simulink model "A320_23b"  (R2023b)
settings: Solver=ode4  StartTime=0.0  StopTime=150  FixedStep=0.001  RelTol=1e-3
InitFcn:
  | % 清空工作区
  | % clear;
  | 
  | % 加载气动数据
  | load('engine_ct_table.mat'); % 或者是你那个存有气动数据的文件名
values from neighbouring files (symbols this model uses):
  a0 = 340.294    [basedata.m]    (also in basedata.mat; control_design.mat; landing_init.m; landing_plan.mat)
  b_ref = 2.0    (= 2)    [basedata.m]    (also in basedata.mat; control_design.mat; landing_init.m; landing_plan.mat)
  c_gear = [0.8e4, 1.4e4, 1.4e4]    [basedata.m]    (also in basedata.mat = [8000 14000 14000]; control_design.mat = [8000 14000 14000]; landing_init.m; landing_plan.mat = [8000 14000 14000])
  c_lat = [1.4e4, 2.2e4, 2.2e4]    [basedata.m]    (also in basedata.mat = [14000 22000 22000]; control_design.mat = [14000 22000 22000]; landing_init.m; landing_plan.mat = [14000 22000 22000])
  c_ref = 0.9    [basedata.m]    (also in basedata.mat; control_design.mat; landing_init.m; landing_plan.mat)
  c_roll = [0.020, 0.018, 0.018]    [basedata.m]    (also in basedata.mat = [0.02 0.018 0.018]; control_design.mat = [0.02 0.018 0.018]; landing_init.m; landing_plan.mat = [0.02 0.018 0.018])
  CD0 = 0.045    [basedata.m]    (also in basedata.mat; canshujisuan.m; control_design.mat; landing_init.m)
  Clb = -0.08    [basedata.m]    (also in basedata.mat; control_design.mat; landing_init.m; landing_plan.mat)
  Clda = -0.20    (= -0.2)    [basedata.m]    (also in basedata.mat; control_design.mat; landing_init.m; landing_plan.mat)
  CLde = 0.28    [basedata.m]    (also in basedata.mat; control_design.mat; landing_init.m; landing_plan.mat)
  Clp = -0.70    (= -0.7)    [basedata.m]    (also in basedata.mat; control_design.mat; landing_init.m; landing_plan.mat)
  CLq = 4.50    (= 4.5)    [basedata.m]    (also in basedata.mat; canshujisuan.m = 3; control_design.mat; landing_init.m)
  Clr = 0.08    [basedata.m]    (also in basedata.mat; control_design.mat; landing_init.m; landing_plan.mat)
  Cmde = -0.90    (= -0.9)    [basedata.m]    (also in basedata.mat; control_design.mat; landing_init.m; landing_plan.mat)
  Cmq = -18.0    (= -18)    [basedata.m]    (also in basedata.mat; control_design.mat; landing_init.m; landing_plan.mat)
  Cnb = 0.25    [basedata.m]    (also in basedata.mat; control_design.mat; landing_init.m; landing_plan.mat)
  Cndr = -0.15    [basedata.m]    (also in basedata.mat; control_design.mat; landing_init.m; landing_plan.mat)
  Cnp = -0.04    [basedata.m]    (also in basedata.mat; control_design.mat; landing_init.m; landing_plan.mat)
  Cnr = -0.45    [basedata.m]    (also in basedata.mat; control_design.mat; landing_init.m; landing_plan.mat)
  CSb = -0.70    (= -0.7)    [basedata.m]    (also in basedata.mat; control_design.mat; landing_init.m; landing_plan.mat)
  CSdr = 0.18    [basedata.m]    (also in basedata.mat; control_design.mat; landing_init.m; landing_plan.mat)
  CSr = 0.12    [basedata.m]    (also in basedata.mat; control_design.mat; landing_init.m; landing_plan.mat)
  D = 0.5 * rho0 * V^2 * S_ref * CD_current    [canshujisuan.m]
  D0 = 1400    [basedata.m]    (also in basedata.mat; control_design.mat = 800; landing.m; landing_init.m)
  da_max = 25    [basedata.m]    (also in basedata.mat; control_design.mat; landing_init.m; landing_plan.mat)
  da_min = -da_max    (= -25)    [basedata.m]    (also in basedata.mat; control_design.mat; landing_init.m; landing_plan.mat)
  de_max = 25    [basedata.m]    (also in basedata.mat; control_design.mat; landing_init.m; landing_plan.mat)
  de_min = -de_max    (= -25)    [basedata.m]    (also in basedata.mat; control_design.mat; landing_init.m; landing_plan.mat)
  DH = pi / 180    (= 0.0174532925199)    [basedata.m]    (also in basedata.mat; control_design.mat; landing_init.m; landing_plan.mat)
  dr_max = 25    [basedata.m]    (also in basedata.mat; control_design.mat; landing_init.m; landing_plan.mat)
  dr_min = -dr_max    (= -25)    [basedata.m]    (also in basedata.mat; control_design.mat; landing_init.m; landing_plan.mat)
  g = 9.80665    [basedata.m]    (also in basedata.mat; canshujisuan.m; control_design.mat; landing_init.m)
  ground_z = 0.0    (= 0)    [basedata.m]    (also in basedata.mat; control_design.mat; landing_init.m; landing_plan.mat)
  H_B = 132.622761894    [basedata.mat]    (also in landing_trajectory.m = H_R - R * cos(a1); landingplan.mat)
  H_C = 72.1000994005    [basedata.mat]    (also in landing_trajectory.m = H_R - R * cos(a2); landingplan.mat)
  H_climb_complete = 1000    [control_design.mat]    (also in landing.m; landing_init.m; landing_plan.mat; landingplan.mat)
  H_entry = 1000    [basedata.mat]    (also in landing_trajectory.m; landingplan.mat)
  H_exp = 20    [basedata.mat]    (also in landing_trajectory.m; landingplan.mat)
  HD = 180 / pi    (= 57.2957795131)    [basedata.m]    (also in basedata.mat; control_design.mat; landing_init.m; landing_plan.mat)
  I = [ Ixx, -Ixy, -Ixz ... (first row only)    [basedata.m]    (also in basedata.mat = [120  0  0; 0  480  0; 0  0  520]; control_design.mat = [120  0  0; 0  480  0; 0  0  520]; landing_init.m; landing_plan.mat = [120  0  0; 0  480  0; 0  0  520])
  K_alpha = 7.5375    [basedata.mat]    (also in control_design.m = (((wd_pitch^2)-a24))/(2*kesi_pitch*wd_pitch); control_design.mat; controller.m = 5; landingplan.mat)
  k_gear = [1.0e5, 3.0e5, 3.0e5]    [basedata.m]    (also in basedata.mat = [100000 300000 300000]; control_design.mat = [100000 300000 300000]; landing_init.m; landing_plan.mat = [100000 300000 300000])
  Kn_pitch = -0.120095403309    [basedata.mat]    (also in control_design.m = -(2.2*g*(wd_pitch)^2)/(Tr*(((wd_pitch)^2)-a24)*V_control*a34; control_design.mat; controller.m = (2.2*wd^2*g)/(Tr*(wd^2-a24)*V_test*a34); landingplan.mat)
  Kw_pitch = -0.483749055178    [basedata.mat]    (also in control_design.m = -2*kesi_pitch*wd_pitch/a25; control_design.mat; controller.m = -(2*zeta*wd) / a25; landingplan.mat)
  m = 600.0    (= 600)    [basedata.m]    (also in basedata.mat; canshujisuan.m; control_design.mat; landing_init.m)
  mu_brake = [0.0, 0.55, 0.55]    [basedata.m]    (also in basedata.mat = [0 0.55 0.55]; control_design.mat = [0 0.55 0.55]; landing_init.m; landing_plan.mat = [0 0.55 0.55])
  phi0 = 0    [control_design.mat]    (also in landing.m; landing_init.m; landing_init.mat; landing_plan.mat)
  psi0 = 0    [control_design.mat]    (also in landing.m; landing_init.m; landing_init.mat; landing_plan.mat)
  r_left_b = r_gear_b(:,2)    [basedata.m]    (also in basedata.mat = [-0.333333333333 -0.8 0.65]; control_design.mat = [-0.333333333333 -0.8 0.65]; landing_init.m; landing_plan.mat = [-0.333333333333 -0.8 0.65])
  r_nose_b = r_gear_b(:,1)    [basedata.m]    (also in basedata.mat = [2 0 0.65]; control_design.mat = [2 0 0.65]; landing_init.m; landing_plan.mat = [2 0 0.65])
  r_right_b = r_gear_b(:,3)    [basedata.m]    (also in basedata.mat = [-0.333333333333 0.8 0.65]; control_design.mat = [-0.333333333333 0.8 0.65]; landing_init.m; landing_plan.mat = [-0.333333333333 0.8 0.65])
  rho0 = 1.225    [basedata.m]    (also in basedata.mat; canshujisuan.m; control_design.mat; landing_init.m)
  S_ref = 1.2    [basedata.m]    (also in basedata.mat; canshujisuan.m; control_design.mat; landing_init.m)
  theta0 = 0    [control_design.mat]    (also in landing.m; landing_init.m; landing_init.mat = 0.0523598775598; landing_plan.mat = 0.0523560209424)
  V_app = 128.516392565    [basedata.mat]    (also in landing_trajectory.m = 1.4 * Vs; landingplan.mat)
  V_cruise = 200    [basedata.m]
  v_eps = 0.20    (= 0.2)    [basedata.m]    (also in basedata.mat; control_design.mat; landing_init.m; landing_plan.mat)
  V_flare = V_shallow    [landing_trajectory.m]
  V_min = 3    [control_design.mat]    (also in landing.m; landing_init.m; landing_plan.mat; landingplan.mat)
  V_shallow = 110.156907913    [basedata.mat]    (also in landing_trajectory.m = 1.2 * Vs; landingplan.mat)
  wheel_radius = 0.18    [basedata.m]    (also in basedata.mat; control_design.mat; landing_init.m; landing_plan.mat)
  WOW_on = 0.000    (= 0)    [basedata.m]    (also in basedata.mat; control_design.mat; landing_init.m; landing_plan.mat)
  Xg0 = 0    [control_design.mat]    (also in landing.m = -12000; landing_init.m = -12000; landing_init.mat = -8000; landing_plan.mat = -12000)
  Yg0 = 3    [control_design.mat]    (also in landing.m = 0; landing_init.m = 0; landing_init.mat = 0; landing_plan.mat = 0)
  Zg0 = ground_z - wheel_radius - r_gear_b(3,1) + static_deflection    [basedata.m]    (also in basedata.mat = -0.8215943; control_design.mat = -0.8215943; landing.m = -1000; landing_init.m = -1000)
undefined symbols (not defined in the file or in its folder): alpha_CL_table, alpha_Cm_table, alpha_Kde_table, CL_D0, CL_table, Cldr, Cm_table, Cnda, CT_ref, CT_table, CYp, Delta_CD_flap_tot, Delta_CD_gear, Delta_CD_sp, Delta_CL_flap_tot, Delta_CL_sp, Delta_Cm_flap_tot, Delta_Cm_gear, Delta_Cm_sp, delta_flap_TE_max, delta_flap_TE_tab, delta_slat_LE_max, delta_slat_LE_tab, gD_flap_TE_tab, gD_slat_LE_tab, gL_flap_TE_tab, gL_slat_LE_tab, I_xz, I_yz, Ix_Iy, Iy_Iz, Iz_Ix, K_GE, k_i_eff, Kde_table, Mach, N1, N1_idle, N1_lim, spoiler_max_air, T_static, X_landing_start
libraries: simulink x51, matrix_library x19
(part 2 of 4)

== system A320_23b/6DOF-MODEL/AERO-PARAMETER/atmosphere ==
  Add : Sum
  Band-Limited White Noise : simulink/Sources/Band-Limited White Noise  Cov=[1]  Ts=0.1  seed=[23341]
  Constant1 : Constant  Value=rho0
  Constant2 : Constant  Value=a0
  Constant3 : Constant  Value=0.5
  Constant4 : Constant  Value=0
  Constant5 : Constant  Value=0
  Constant6 : Constant  Value=5
  Display : Display
  Gain : Gain
  MATLAB Function : MATLAB Function  TreatAsAtomicUnit=on
  Matrix Multiply : Product  Multiplication=Matrix(*)
  Mux : Mux  Inputs=3
  Product : Product  Inputs=3
  Reshape : Reshape  OutputDimensionality=Column vector (2-D)
  Scope : Scope
  Square : Math  Operator=square
  Transfer Fcn : TransferFcn  Denominator=[10 1]
  tag scope: Vwind_body=global, Vwind_ground=global, a_sound=global, qc=global, rho=global
  wires:
  Constant1/1 -> [rho]
  Constant2/1 -> [a_sound]
  Constant3/1 -> Product/1
  [rho] -> Product/2
  Product/1 -> Display/1, [qc]
  Square/1 -> Product/3
  [Vg] -> Square/1
  Reshape/1 -> [Vwind_ground]
  [Vwind_ground] -> Matrix Multiply/2
  [theta_eular] -> MATLAB Function/2(theta)
  [phi_eular] -> MATLAB Function/1(phi)
  MATLAB Function/1(R_bg) -> Matrix Multiply/1
  [psi_eular] -> MATLAB Function/3(psi)
  Matrix Multiply/1 -> [Vwind_body]
  Gain/1 -> Add/1
  Transfer Fcn/1 -> Gain/1
  Band-Limited White Noise/1 -> Transfer Fcn/1
  Constant5/1 -> Mux/3
  Constant4/1 -> Mux/1
  Add/1 -> Scope/1, Mux/2
  Constant6/1 -> Add/2

== system A320_23b/6DOF-MODEL/AERO-PARAMETER/侧向力系数 ==
  beta(H) : Inport
  dr(H) : Inport  Port=2
  Add : Sum  Inputs=++++
  CYpConst : Constant  Value=CYp
  CYpXPhat : Product
  Constant1 : Constant  Value=CSb
  Constant2 : Constant  Value=CSr
  Constant3 : Constant  Value=CSdr
  Product : Product
  Product2 : Product
  Product3 : Product
  CS : Outport
  wires:
  Add/1 -> CS/1
  Constant3/1 -> Product2/2
  Product2/1 -> Add/3
  dr(H)/1 -> Product2/1
  beta(H)/1 -> Product/1
  Constant1/1 -> Product/2
  Constant2/1 -> Product3/2
  [r_hat] -> Product3/1
  Product/1 -> Add/1
  Product3/1 -> Add/2
  [p_hat] -> CYpXPhat/1
  CYpConst/1 -> CYpXPhat/2
  CYpXPhat/1 -> Add/4

== system A320_23b/6DOF-MODEL/AERO-PARAMETER/俯仰力矩系数 ==
  alpha(H) : Inport
  de(H) : Inport  Port=2
  delta_flap_TE : Inport  Port=3
  delta_slat_LE : Inport  Port=4
  delta_spL : Inport  Port=5
  delta_spR : Inport  Port=6
  eta_gear : Inport  Port=7
  Add : Sum  Inputs=++++++
  CmdeXKde : Product
  Constant1 : Lookup_n-D  NumberOfTableDimensions=1  BreakpointsForDimension1=alpha_Cm_table  Table=Cm_table  InterpMethod=Akima spline
  Constant2 : Constant  Value=Cmq
  Constant3 : Constant  Value=Cmde
  FlapMSum : Sum  Inputs=|++
  FlapMTotal : Gain  Gain=Delta_Cm_flap_tot
  Gain : Gain  Gain=-1
  GearMTotal : Gain  Gain=Delta_Cm_gear
  KdeLookup : Lookup_n-D  NumberOfTableDimensions=1  BreakpointsForDimension1=alpha_Kde_table  Table=Kde_table  InterpMethod=Akima spline
  LENorm : Gain  Gain=1/delta_slat_LE_max
  Product2 : Product
  Product3 : Product
  SpMEta : Gain  Gain=1/(2*spoiler_max_air)
  SpMSum : Sum  Inputs=|++
  SpMTotal : Gain  Gain=Delta_Cm_sp
  TENorm : Gain  Gain=1/delta_flap_TE_max
  Cm : Outport
  wires:
  de(H)/1 -> Product2/1
  Add/1 -> Cm/1
  Constant2/1 -> Product3/2
  [q_hat] -> Product3/1
  Product3/1 -> Add/3
  alpha(H)/1 -> KdeLookup/1, Constant1/1
  Constant3/1 -> CmdeXKde/1
  KdeLookup/1 -> CmdeXKde/2
  CmdeXKde/1 -> Product2/2
  Constant1/1 -> Gain/1
  delta_flap_TE/1 -> TENorm/1
  delta_slat_LE/1 -> LENorm/1
  TENorm/1 -> FlapMSum/1
  LENorm/1 -> FlapMSum/2
  FlapMSum/1 -> FlapMTotal/1
  FlapMTotal/1 -> Add/5
  delta_spL/1 -> SpMSum/1
  delta_spR/1 -> SpMSum/2
  SpMSum/1 -> SpMEta/1
  SpMEta/1 -> SpMTotal/1
  SpMTotal/1 -> Add/6
  eta_gear/1 -> GearMTotal/1
  GearMTotal/1 -> Add/4
  Product2/1 -> Add/2
  Gain/1 -> Add/1

== system A320_23b/6DOF-MODEL/AERO-PARAMETER/偏航力矩系数 ==
  beta(H) : Inport
  dr(H) : Inport  Port=2
  da(H) : Inport  Port=3
  Add : Sum  Inputs=+++++
  CndaConst : Constant  Value=Cnda
  CndaXDa : Product
  Constant1 : Constant  Value=Cnb
  Constant2 : Constant  Value=Cnp
  Constant3 : Constant  Value=Cndr
  Constant4 : Constant  Value=Cnr
  Product{,1..3} (4 alike) : Product
  Cn : Outport
  wires:
  Product2/1 -> Add/4
  Constant4/1 -> Product1/2
  Product/1 -> Add/1
  dr(H)/1 -> Product2/1
  Constant3/1 -> Product2/2
  beta(H)/1 -> Product/1
  Constant1/1 -> Product/2
  Add/1 -> Cn/1
  Constant2/1 -> Product3/2
  [p_hat] -> Product3/1
  Product1/1 -> Add/3
  [r_hat] -> Product1/1
  Product3/1 -> Add/2
  da(H)/1 -> CndaXDa/1
  CndaConst/1 -> CndaXDa/2
  CndaXDa/1 -> Add/5

== system A320_23b/6DOF-MODEL/AERO-PARAMETER/力矩系数2力矩 ==
  Cl/Cm/Cn : Inport
  Constant : Constant  Value=S_ref
  Constant1 : Constant  Value=c_ref
  Constant2 : Constant  Value=b_ref
  Demux : Demux  Outputs=3
  Mux : Mux  Inputs=3
  Product : Product  Inputs=4
  Product1 : Product  Inputs=4
  Product2 : Product  Inputs=4
  MX/MY/MZ : Outport
  wires:
  Cl/Cm/Cn/1 -> Demux/1
  Demux/1 -> Product/1
  Constant/1 -> Product/2, Product1/2, Product2/2
  Demux/3 -> Product2/1
  Demux/2 -> Product1/1
  [qc] -> Product/3, Product2/3, Product1/3
  Product/1 -> Mux/1
  Product1/1 -> Mux/2
  Product2/1 -> Mux/3
  Mux/1 -> MX/MY/MZ/1
  Constant2/1 -> Product/4, Product2/4
  Constant1/1 -> Product1/4

== system A320_23b/6DOF-MODEL/AERO-PARAMETER/力系数2力 ==
  CD/CL/CS : Inport
  Constant : Constant  Value=S_ref
  Demux : Demux  Outputs=3
  Display : Display
  Display1 : Display
  Display2 : Display
  Gain : Gain  Gain=-1
  Gain1 : Gain  Gain=-1
  Mux : Mux  Inputs=3
  Product : Product  Inputs=3
  Product1 : Product  Inputs=3
  Product2 : Product  Inputs=3
  D/L/S : Outport
  wires:
  CD/CL/CS/1 -> Demux/1
  Demux/1 -> Product/1
  Constant/1 -> Product2/2, Product1/2, Product/2
  Demux/3 -> Product2/1
  Demux/2 -> Product1/1
  [qc] -> Product2/3, Product1/3, Product/3
  Product/1 -> Display/1, Gain/1
  Product1/1 -> Display1/1, Gain1/1
  Product2/1 -> Display2/1, Mux/3
  Mux/1 -> D/L/S/1
  Gain/1 -> Mux/1
  Gain1/1 -> Mux/2

== system A320_23b/6DOF-MODEL/AERO-PARAMETER/升力系数 ==
  alpha(H) : Inport
  de(H) : Inport  Port=2
  delta_flap_TE : Inport  Port=3
  delta_slat_LE : Inport  Port=4
  delta_spL : Inport  Port=5
  delta_spR : Inport  Port=6
  Add : Sum  Inputs=+++++
  Constant1 : Lookup_n-D  NumberOfTableDimensions=1  BreakpointsForDimension1=alpha_CL_table  Table=CL_table  InterpMethod=Akima spline
  Constant2 : Constant  Value=CLq
  Constant3 : Constant  Value=CLde
  FlapSum : Sum  Inputs=|++
  FlapTotal : Gain  Gain=Delta_CL_flap_tot
  GLLELkup : Lookup_n-D  NumberOfTableDimensions=1  BreakpointsForDimension1=delta_slat_LE_tab  Table=gL_slat_LE_tab  InterpMethod=Akima spline
  GLTELkup : Lookup_n-D  NumberOfTableDimensions=1  BreakpointsForDimension1=delta_flap_TE_tab  Table=gL_flap_TE_tab  InterpMethod=Akima spline
  KGEGain : Gain  Gain=K_GE
  Product2 : Product
  Product3 : Product
  SlatW : Gain  Gain=0.01
  SpEta : Gain  Gain=1/(2*spoiler_max_air)
  SpSum : Sum  Inputs=|++
  SpTotal : Gain  Gain=Delta_CL_sp
  CL : Outport
  tag scope: CLa=global
  wires:
  [q_hat] -> Product3/1
  Constant2/1 -> Product3/2
  de(H)/1 -> Product2/1
  Constant3/1 -> Product2/2
  Product2/1 -> Add/4
  Product3/1 -> Add/3
  alpha(H)/1 -> Constant1/1
  Constant1/1 -> [CLa], Add/1
  Add/1 -> KGEGain/1
  KGEGain/1 -> CL/1
  delta_flap_TE/1 -> GLTELkup/1
  delta_slat_LE/1 -> GLLELkup/1
  GLTELkup/1 -> FlapSum/1
  GLLELkup/1 -> SlatW/1
  SlatW/1 -> FlapSum/2
  FlapSum/1 -> FlapTotal/1
  delta_spL/1 -> SpSum/1
  delta_spR/1 -> SpSum/2
  SpSum/1 -> SpEta/1
  SpEta/1 -> SpTotal/1
  FlapTotal/1 -> Add/2
  SpTotal/1 -> Add/5

== system A320_23b/6DOF-MODEL/AERO-PARAMETER/无量纲化角速率 ==
  p : Inport
  q : Inport  Port=2
  r : Inport  Port=3
  Constant : Constant  Value=V_min
  Max : MinMax  Function=max  Inputs=2
  Scope : Scope
  Subsystem : Subsystem
  Subsystem1 : Subsystem
  Subsystem2 : Subsystem
  tag scope: Va_safe=global, p_hat=global, q_hat=global, r_hat=global
  wires:
  p/1 -> Subsystem2/1(p)
  [Va_safe] -> Subsystem2/2(Va), Subsystem1/2(Va), Subsystem/2(Va)
  Subsystem/1(r_hat) -> [r_hat]
  Subsystem1/1(q_hat) -> Scope/1, [q_hat]
  Subsystem2/1(p_hat) -> [p_hat]
  [Va] -> Max/2
  Constant/1 -> Max/1
  Max/1 -> [Va_safe]
  r/1 -> Subsystem/1(r)
  q/1 -> Subsystem1/1(q)

== system A320_23b/6DOF-MODEL/AERO-PARAMETER/滚转力矩系数 ==
  beta(H) : Inport
  da(H) : Inport  Port=2
  dr(H) : Inport  Port=3
  Add : Sum  Inputs=+++++
  CldrConst : Constant  Value=Cldr
  CldrXDr : Product
  Constant1 : Constant  Value=Clb
  Constant2 : Constant  Value=Clp
  Constant3 : Constant  Value=Clda
  Constant4 : Constant  Value=Clr
  Product{,1..3} (4 alike) : Product
  Cl : Outport
  wires:
  Product3/1 -> Add/2
  da(H)/1 -> Product2/1
  Product/1 -> Add/1
  beta(H)/1 -> Product/1
  Add/1 -> Cl/1
  Constant1/1 -> Product/2
  Constant3/1 -> Product2/2
  Constant2/1 -> Product3/2
  [p_hat] -> Product3/1
  Product1/1 -> Add/3
  [r_hat] -> Product1/1
  Constant4/1 -> Product1/2
  Product2/1 -> Add/4
  dr(H)/1 -> CldrXDr/1
  CldrConst/1 -> CldrXDr/2
  CldrXDr/1 -> Add/5

== system A320_23b/6DOF-MODEL/AERO-PARAMETER/阻力系数 ==
  delta_flap_TE : Inport
  delta_slat_LE : Inport  Port=2
  delta_spL : Inport  Port=3
  delta_spR : Inport  Port=4
  eta_gear : Inport  Port=5
  Add : Sum  Inputs=+++++
  CLD0Cfg : Constant  Value=CL_D0
  CLSub : Sum  Inputs=+-
  Constant : Constant  Value=CD0
  Constant1 : Constant  Value=k_i_eff
  FlapDSum : Sum  Inputs=|++
  FlapDTotal : Gain  Gain=Delta_CD_flap_tot
  GDLELkup : Lookup_n-D  NumberOfTableDimensions=1  BreakpointsForDimension1=delta_slat_LE_tab  Table=gD_slat_LE_tab  InterpMethod=Akima spline
  GDTELkup : Lookup_n-D  NumberOfTableDimensions=1  BreakpointsForDimension1=delta_flap_TE_tab  Table=gD_flap_TE_tab  InterpMethod=Akima spline
  GearDTotal : Gain  Gain=Delta_CD_gear
  LEDWeight : Gain  Gain=0.5
  Product : Product
  SpDEta : Gain  Gain=1/(2*spoiler_max_air)
  SpDSum : Sum  Inputs=|++
  SpDTotal : Gain  Gain=Delta_CD_sp
  Square : Math  Operator=square
  CD : Outport
  wires:
  Constant/1 -> Add/1
  Constant1/1 -> Product/1
  Square/1 -> Product/2
  Product/1 -> Add/2
  Add/1 -> CD/1
  [CL] -> CLSub/1
  CLD0Cfg/1 -> CLSub/2
  CLSub/1 -> Square/1
  delta_flap_TE/1 -> GDTELkup/1
  delta_slat_LE/1 -> GDLELkup/1
  GDLELkup/1 -> LEDWeight/1
  GDTELkup/1 -> FlapDSum/1
  LEDWeight/1 -> FlapDSum/2
  FlapDSum/1 -> FlapDTotal/1
  delta_spL/1 -> SpDSum/1
  delta_spR/1 -> SpDSum/2
  SpDSum/1 -> SpDEta/1
  SpDEta/1 -> SpDTotal/1
  eta_gear/1 -> GearDTotal/1
  FlapDTotal/1 -> Add/3
  GearDTotal/1 -> Add/4
  SpDTotal/1 -> Add/5

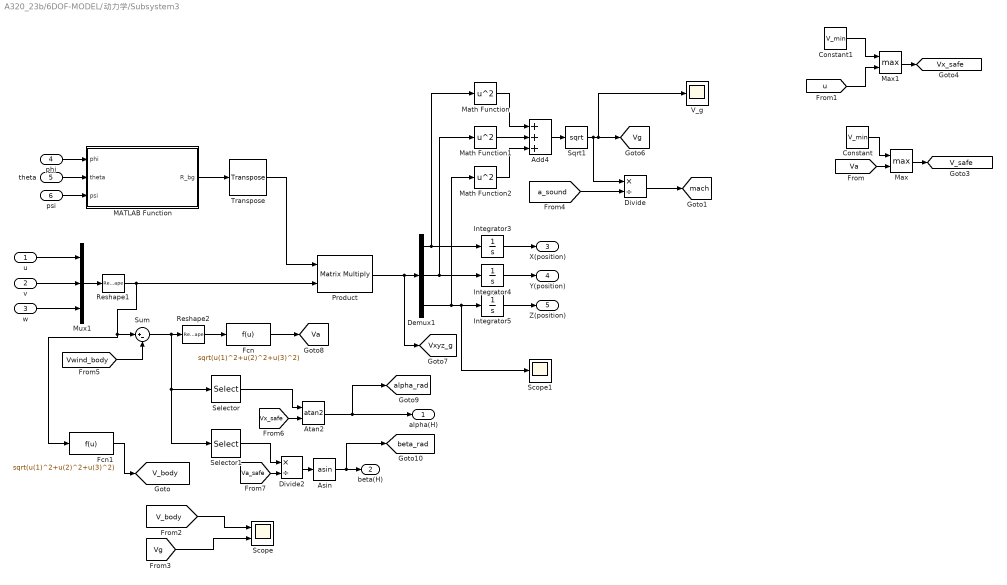
== system A320_23b/6DOF-MODEL/动力学/Subsystem3 ==
  u : Inport
  v : Inport  Port=2
  w : Inport  Port=3
  phi : Inport  Port=4
  theta : Inport  Port=5
  psi : Inport  Port=6
  Add4 : Sum  Inputs=+++
  Asin : Trigonometry  Operator=asin
  Atan2 : Trigonometry  Operator=atan2
  Constant : Constant  Value=V_min
  Constant1 : Constant  Value=V_min  VectorParams1D=off
  Demux1 : Demux  Outputs=3
  Divide : Product  Inputs=*/
  Divide2 : Product  Inputs=*/
  Fcn : Fcn  Expr=sqrt(u(1)^2+u(2)^2+u(3)^2)
  Fcn1 : Fcn  Expr=sqrt(u(1)^2+u(2)^2+u(3)^2)
  Integrator3 : Integrator  InitialCondition=Xg0
  Integrator4 : Integrator  InitialCondition=Yg0
  Integrator5 : Integrator  InitialCondition=Zg0
  MATLAB Function : MATLAB Function  TreatAsAtomicUnit=on
  Math Function : Math  Operator=square
  Math Function1 : Math  Operator=square
  Math Function2 : Math  Operator=square
  Max : MinMax  Function=max  Inputs=2
  Max1 : MinMax  Function=max  Inputs=2
  Mux1 : Mux  Inputs=3
  Product : Product  Multiplication=Matrix(*)
  Reshape1 : Reshape  OutputDimensionality=Column vector (2-D)
  Reshape2 : Reshape
  Scope : Scope  NumInputPorts=2
  Scope1 : Scope
  Selector : Selector  InputPortWidth=3  IndexOptions=Index vector (dialog)  Indices=3  OutputSizes=1
  Selector1 : Selector  InputPortWidth=3  IndexOptions=Index vector (dialog)  Indices=2  OutputSizes=1
  Sqrt1 : Sqrt
  Sum : Sum  Inputs=|+-
  Transpose : matrix_library/Transpose
  V_g : Scope
  alpha(H) : Outport
  beta(H) : Outport  Port=2
  X(position) : Outport  Port=3
  Y(position) : Outport  Port=4
  Z(position) : Outport  Port=5
  tag scope: V_body=global, V_safe=global, Va=global, Vg=global, Vx_safe=global, Vxyz_g=global, alpha_rad=global, beta_rad=global, mach=global
  wires:
  Constant/1 -> Max/1
  Max/1 -> [V_safe]
  [Va] -> Max/2
  Constant1/1 -> Max1/1
  Max1/1 -> [Vx_safe]
  [u] -> Max1/2
  phi/1 -> MATLAB Function/1(phi)
  Demux1/2 -> Math Function1/1, Integrator4/1
  Demux1/1 -> Math Function/1, Integrator3/1
  Fcn/1 -> [Va]
  Product/1 -> [Vxyz_g], Demux1/1
  Mux1/1 -> Reshape1/1
  theta/1 -> MATLAB Function/2(theta)
  u/1 -> Mux1/1
  Math Function2/1 -> Add4/3
  Reshape2/1 -> Fcn/1
  v/1 -> Mux1/2
  Demux1/3 -> Math Function2/1, Scope1/1, Integrator5/1
  MATLAB Function/1(R_bg) -> Transpose/1
  Sum/1 -> Selector1/1, Selector/1, Reshape2/1
  Add4/1 -> Sqrt1/1
  Math Function/1 -> Add4/1
  Math Function1/1 -> Add4/2
  psi/1 -> MATLAB Function/3(psi)
  Atan2/1 -> [alpha_rad], alpha(H)/1
  Reshape1/1 -> Fcn1/1, Sum/1, Product/2
  Transpose/1 -> Product/1
  w/1 -> Mux1/3
  Integrator3/1 -> X(position)/1
  Integrator4/1 -> Y(position)/1
  Integrator5/1 -> Z(position)/1
  [Vwind_body] -> Sum/2
  [Vx_safe] -> Atan2/2
  Selector/1 -> Atan2/1
  [Va_safe] -> Divide2/2
  Selector1/1 -> Divide2/1
  Divide2/1 -> Asin/1
  Asin/1 -> [beta_rad], beta(H)/1
  Fcn1/1 -> [V_body]
  [V_body] -> Scope/1
  [Vg] -> Scope/2
  Sqrt1/1 -> Divide/1, [Vg], V_g/1
  [a_sound] -> Divide/2
  Divide/1 -> [mach]

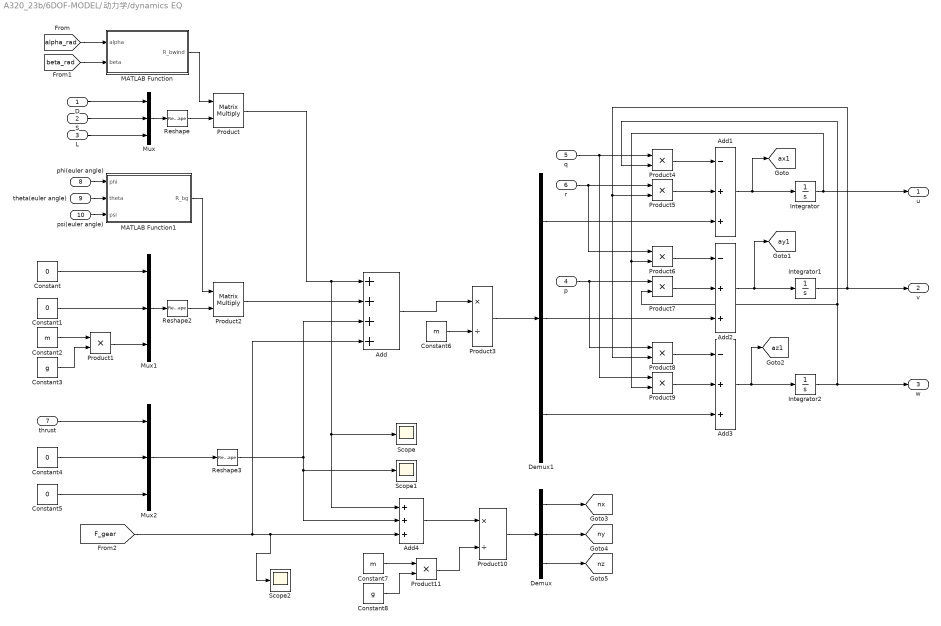
== system A320_23b/6DOF-MODEL/动力学/dynamics EQ ==
  D : Inport
  S : Inport  Port=2
  L : Inport  Port=3
  p : Inport  Port=4
  q : Inport  Port=5
  r : Inport  Port=6
  thrust : Inport  Port=7
  phi(euler angle) : Inport  Port=8
  theta(euler angle) : Inport  Port=9
  psi(euler angle) : Inport  Port=10
  Add : Sum  Inputs=++++
  Add1 : Sum  Inputs=-++
  Add2 : Sum  Inputs=-++
  Add3 : Sum  Inputs=-++
  Add4 : Sum  Inputs=+++
  Constant{,1,4..5} (4 alike) : Constant  Value=0
  Constant2 : Constant  Value=m
  Constant3 : Constant  Value=g
  Constant6 : Constant  Value=m
  Constant7 : Constant  Value=m
  Constant8 : Constant  Value=g
  Demux : Demux  Outputs=3
  Demux1 : Demux  Outputs=3
  Integrator : Integrator  InitialCondition=200
  Integrator1 : Integrator
  Integrator2 : Integrator
  MATLAB Function : MATLAB Function  TreatAsAtomicUnit=on
  MATLAB Function1 : MATLAB Function  TreatAsAtomicUnit=on
  Mux : Mux  Inputs=3
  Mux1 : Mux  Inputs=3
  Mux2 : Mux  Inputs=3
  Product : Product  Multiplication=Matrix(*)
  Product{1,4..9,11} (8 alike) : Product
  Product10 : Product  Inputs=*/
  Product2 : Product  Multiplication=Matrix(*)
  Product3 : Product  Inputs=*/
  Reshape : Reshape  OutputDimensionality=Column vector (2-D)
  Reshape2 : Reshape  OutputDimensionality=Column vector (2-D)
  Reshape3 : Reshape  OutputDimensionality=Column vector (2-D)
  Scope : Scope
  Scope1 : Scope
  Scope2 : Scope
  u : Outport
  v : Outport  Port=2
  w : Outport  Port=3
  tag scope: ax1=global, ay1=global, az1=global, nx=global, ny=global, nz=global
  wires:
  S/1 -> Mux/2
  D/1 -> Mux/1
  L/1 -> Mux/3
  Mux/1 -> Reshape/1
  Reshape/1 -> Product/2
  MATLAB Function/1(R_bwind) -> Product/1
  thrust/1 -> Mux2/1
  theta(euler angle)/1 -> MATLAB Function1/2(theta)
  phi(euler angle)/1 -> MATLAB Function1/1(phi)
  psi(euler angle)/1 -> MATLAB Function1/3(psi)
  Constant2/1 -> Product1/1
  Constant3/1 -> Product1/2
  Constant1/1 -> Mux1/2
  Constant/1 -> Mux1/1
  Product1/1 -> Mux1/3
  Mux1/1 -> Reshape2/1
  Reshape2/1 -> Product2/2
  Constant4/1 -> Mux2/2
  Constant5/1 -> Mux2/3
  Mux2/1 -> Reshape3/1
  Add/1 -> Product3/1
  Product3/1 -> Demux1/1
  Add1/1 -> Integrator/1, [ax1]
  MATLAB Function1/1(R_bg) -> Product2/1
  Product2/1 -> Add/2
  Reshape3/1 -> Add4/2, Scope1/1, Add/3
  Product/1 -> Add/1, Add4/1, Scope/1
  Constant6/1 -> Product3/2
  Demux1/1 -> Add1/3
  Product5/1 -> Add1/2
  r/1 -> Product6/1, Product5/1
  q/1 -> Product9/1, Product4/1
  Demux1/2 -> Add2/3
  Product7/1 -> Add2/2
  Product4/1 -> Add1/1
  Product6/1 -> Add2/1
  Product8/1 -> Add3/1
  Product9/1 -> Add3/2
  Demux1/3 -> Add3/3
  p/1 -> Product8/1, Product7/1
  Integrator/1 -> Product6/2, Product9/2, u/1
  Add2/1 -> [ay1], Integrator1/1
  Integrator1/1 -> Product8/2, Product5/2, v/1
  Add3/1 -> [az1], Integrator2/1
  Integrator2/1 -> Product7/2, Product4/2, w/1
  Add4/1 -> Product10/1
  Product11/1 -> Product10/2
  Constant8/1 -> Product11/2
  Constant7/1 -> Product11/1
  Product10/1 -> Demux/1
  Demux/1 -> [nx]
  Demux/2 -> [ny]
  Demux/3 -> [nz]
  [alpha_rad] -> MATLAB Function/1(alpha)
  [beta_rad] -> MATLAB Function/2(beta)
  [F_gear] -> Scope2/1, Add4/3, Add/4

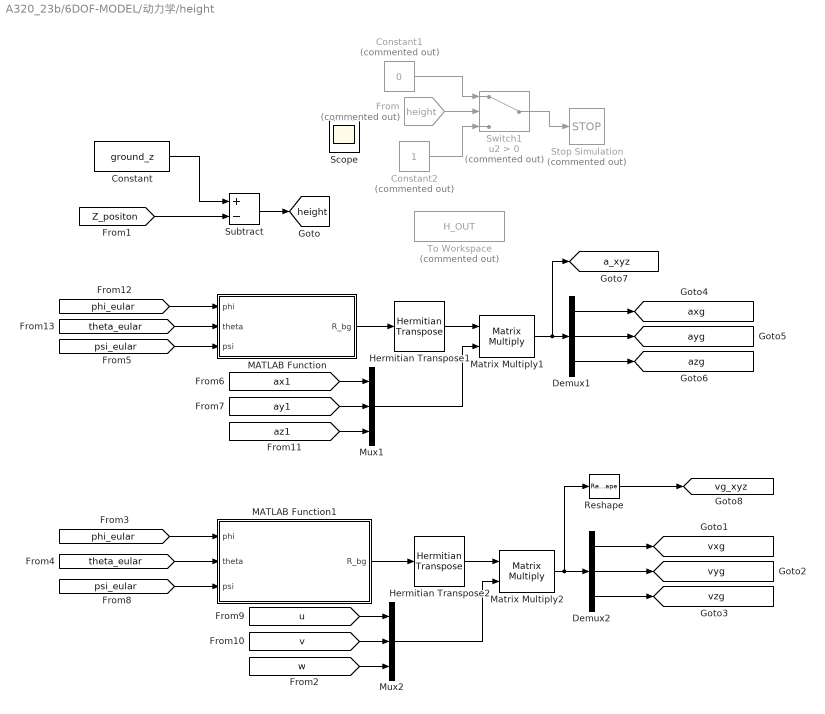
== system A320_23b/6DOF-MODEL/动力学/height ==
  Constant : Constant  Value=ground_z
  Constant1 : Constant  Commented=on  Value=0
  Constant2 : Constant  Commented=on
  Demux1 : Demux  Outputs=3
  Demux2 : Demux  Outputs=3
  From : From  Commented=on  GotoTag=height  TagVisibility=global
  Hermitian Transpose1 : matrix_library/Hermitian Transpose
  Hermitian Transpose2 : matrix_library/Hermitian Transpose
  MATLAB Function : MATLAB Function  TreatAsAtomicUnit=on
  MATLAB Function1 : MATLAB Function  TreatAsAtomicUnit=on
  Matrix Multiply1 : Product  Multiplication=Matrix(*)
  Matrix Multiply2 : Product  Multiplication=Matrix(*)
  Mux1 : Mux  Inputs=3
  Mux2 : Mux  Inputs=3
  Reshape : Reshape  OutputDimensionality=Customize  OutputDimensions=[3,1]
  Scope : Scope
  Stop Simulation : Stop  Commented=on
  Subtract : Sum  Inputs=+-
  Switch1 : Switch  Commented=on  Criteria=u2 > Threshold  SaturateOnIntegerOverflow=off  InputSameDT=off
  To Workspace : ToWorkspace  Commented=on  VariableName=H_OUT  SaveFormat=Timeseries  SampleTime=-1
  tag scope: a_xyz=global, axg=global, ayg=global, azg=global, height=global, vg_xyz=global, vxg=global, vyg=global, vzg=global
  wires:
  [ax1] -> Mux1/1
  [theta_eular] -> MATLAB Function/2(theta)
  MATLAB Function/1(R_bg) -> Hermitian Transpose1/1
  [psi_eular] -> MATLAB Function/3(psi)
  [ay1] -> Mux1/2
  Mux1/1 -> Matrix Multiply1/2
  [phi_eular] -> MATLAB Function/1(phi)
  Matrix Multiply1/1 -> [a_xyz], Demux1/1
  [az1] -> Mux1/3
  Demux1/3 -> [azg]
  Demux1/1 -> [axg]
  Demux1/2 -> [ayg]
  Hermitian Transpose1/1 -> Matrix Multiply1/1
  Switch1/1 -> Stop Simulation/1
  From/1 -> Switch1/2
  Constant1/1 -> Switch1/1
  Constant2/1 -> Switch1/3
  Demux2/2 -> [vyg]
  [u] -> Mux2/1
  Demux2/3 -> [vzg]
  [w] -> Mux2/3
  Mux2/1 -> Matrix Multiply2/2
  [phi_eular] -> MATLAB Function1/1(phi)
  Matrix Multiply2/1 -> Reshape/1, Demux2/1
  Hermitian Transpose2/1 -> Matrix Multiply2/1
  [v] -> Mux2/2
  [theta_eular] -> MATLAB Function1/2(theta)
  [psi_eular] -> MATLAB Function1/3(psi)
  Demux2/1 -> [vxg]
  MATLAB Function1/1(R_bg) -> Hermitian Transpose2/1
  [Z_positon] -> Subtract/2
  Constant/1 -> Subtract/1
  Subtract/1 -> [height]
  Reshape/1 -> [vg_xyz]

== system A320_23b/6DOF-MODEL/动力学/rotation EQ ==
  L : Inport
  M : Inport  Port=2
  N : Inport  Port=3
  Constant : Constant  Value=I
  Demux : Demux  Outputs=3
  Display3 : Display
  Gain : Gain  Gain=inv(I)  Multiplication=Matrix(K*u) (u vector)
  Integrator : Integrator
  Integrator1 : Integrator
  Integrator2 : Integrator
  MATLAB Function1 : MATLAB Function  TreatAsAtomicUnit=on
  Mux : Mux  Inputs=3
  Mux1 : Mux  Inputs=3
  Product : Product  Inputs=3  Multiplication=Matrix(*)
  Reshape : Reshape  OutputDimensionality=Column vector (2-D)
  Reshape1 : Reshape
  Reshape2 : Reshape  OutputDimensionality=Column vector (2-D)
  Subsystem3 : Subsystem  Commented=on
  Sum : Sum  Inputs=|+-
  Sum1 : Sum  Inputs=|++
  p : Outport  VectorParamsAs1DForOutWhenUnconnected=off
  q : Outport  Port=2  VectorParamsAs1DForOutWhenUnconnected=off
  r : Outport  Port=3  VectorParamsAs1DForOutWhenUnconnected=off
  wires:
  Mux/1 -> Reshape/1, Display3/1
  Sum/1 -> Gain/1
  Demux/1 -> Integrator/1
  Demux/2 -> Integrator2/1
  Demux/3 -> Integrator1/1
  Gain/1 -> Reshape1/1
  Reshape1/1 -> Demux/1
  N/1 -> Mux/3
  L/1 -> Mux/1
  M/1 -> Mux/2
  Product/1 -> Sum/2
  MATLAB Function1/1(wB_X) -> Product/1
  Constant/1 -> Product/2
  Integrator/1 -> p/1, Mux1/1
  Integrator1/1 -> r/1, Mux1/3
  Integrator2/1 -> q/1, Mux1/2
  Reshape2/1 -> Product/3
  Mux1/1 -> Reshape2/1, MATLAB Function1/1(w)
  Reshape/1 -> Sum1/1
  [M_gear] -> Sum1/2
  Sum1/1 -> Sum/1

== system A320_23b/6DOF-MODEL/动力学/姿态角 ==
  p : Inport
  q : Inport  Port=2
  r : Inport  Port=3
  Subsystem : Subsystem
  Subsystem1 : Subsystem
  Subsystem2 : Subsystem
  phi(eular) : Outport
  theta(eular) : Outport  Port=2
  psi(eular) : Outport  Port=3
  tag scope: phi_eular=global, psi_eular=global, theta_eular=global
  wires:
  q/1 -> Subsystem2/1(q), Subsystem1/1(q), Subsystem/2(q)
  Subsystem2/1(psi(euler)) -> [psi_eular], psi(eular)/1
  r/1 -> Subsystem2/2(r), Subsystem1/2(r), Subsystem/3(r)
  Subsystem/1(phi(euler)) -> Subsystem1/3(phi(euler)), Subsystem2/3(phi(euler)), phi(eular)/1, [phi_eular]
  Subsystem1/1(theta(euler)) -> Subsystem/4(theta(euler)), theta(eular)/1, [theta_eular], Subsystem2/4(theta(euler))
  p/1 -> Subsystem/1(p)

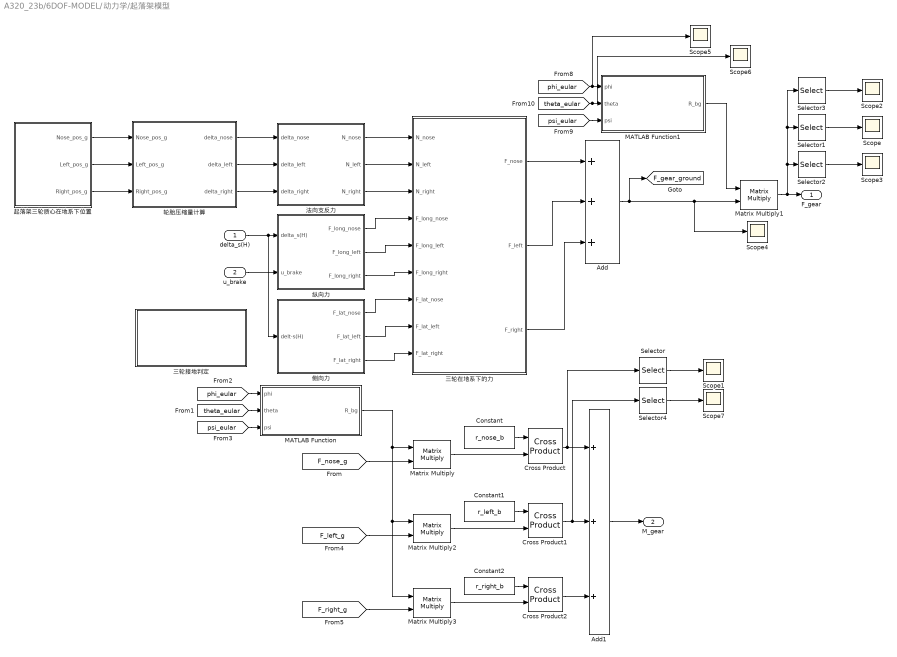
== system A320_23b/6DOF-MODEL/动力学/起落架模型 ==
  delta_s(H) : Inport
  u_brake : Inport  Port=2
  Add : Sum  Inputs=+++
  Add1 : Sum  Inputs=+++
  Constant : Constant  Value=r_nose_b
  Constant1 : Constant  Value=r_left_b
  Constant2 : Constant  Value=r_right_b
  Cross Product : matrix_library/Cross Product
  Cross Product1 : matrix_library/Cross Product
  Cross Product2 : matrix_library/Cross Product
  MATLAB Function : MATLAB Function  TreatAsAtomicUnit=on
  MATLAB Function1 : MATLAB Function  TreatAsAtomicUnit=on
  Matrix Multiply{,1..3} (4 alike) : Product  Multiplication=Matrix(*)
  Scope{,1..7} (8 alike) : Scope
  Selector : Selector  InputPortWidth=3  IndexOptions=Index vector (dialog)  Indices=3  OutputSizes=1
  Selector1 : Selector  InputPortWidth=3  IndexOptions=Index vector (dialog)  Indices=2  OutputSizes=1
  Selector2 : Selector  InputPortWidth=3  IndexOptions=Index vector (dialog)  Indices=3  OutputSizes=1
  Selector3 : Selector  InputPortWidth=3  IndexOptions=Index vector (dialog)  Indices=1  OutputSizes=1
  Selector4 : Selector  InputPortWidth=3  IndexOptions=Index vector (dialog)  Indices=3  OutputSizes=1
  三轮在地系下的力 : Subsystem
  三轮接地判定 : Subsystem
  侧向力 : Subsystem
  法向支反力 : Subsystem
  纵向力 : Subsystem
  起落架三轮质心在地系下位置 : Subsystem
  轮胎压缩量计算 : Subsystem
  F_gear : Outport
  M_gear : Outport  Port=2
  tag scope: F_gear_ground=global
  wires:
  起落架三轮质心在地系下位置/1(Nose_pos_g) -> 轮胎压缩量计算/1(Nose_pos_g)
  起落架三轮质心在地系下位置/2(Left_pos_g) -> 轮胎压缩量计算/2(Left_pos_g)
  起落架三轮质心在地系下位置/3(Right_pos_g) -> 轮胎压缩量计算/3(Right_pos_g)
  轮胎压缩量计算/1(delta_nose) -> 法向支反力/1(delta_nose)
  轮胎压缩量计算/2(delta_left) -> 法向支反力/2(delta_left)
  轮胎压缩量计算/3(delta_right) -> 法向支反力/3(delta_right)
  delta_s(H)/1 -> 侧向力/1(delt-s(H)), 纵向力/1(delta_s(H))
  u_brake/1 -> 纵向力/2(u_brake)
  法向支反力/1(N_nose) -> 三轮在地系下的力/1(N_nose)
  法向支反力/2(N_left) -> 三轮在地系下的力/2(N_left)
  法向支反力/3(N_right) -> 三轮在地系下的力/3(N_right)
  纵向力/1(F_long_nose) -> 三轮在地系下的力/4(F_long_nose)
  纵向力/2(F_long_left) -> 三轮在地系下的力/5(F_long_left)
  纵向力/3(F_long_right) -> 三轮在地系下的力/6(F_long_right)
  侧向力/1(F_lat_nose) -> 三轮在地系下的力/7(F_lat_nose)
  侧向力/2(F_lat_left) -> 三轮在地系下的力/8(F_lat_left)
  侧向力/3(F_lat_right) -> 三轮在地系下的力/9(F_lat_right)
  三轮在地系下的力/1(F_nose) -> Add/1
  三轮在地系下的力/2(F_left) -> Add/2
  三轮在地系下的力/3(F_right) -> Add/3
  Add/1 -> Scope4/1, Matrix Multiply1/2, [F_gear_ground]
  MATLAB Function1/1(R_bg) -> Matrix Multiply1/1
  [phi_eular] -> MATLAB Function1/1(phi), Scope5/1
  Matrix Multiply1/1 -> Selector3/1, Selector1/1, Selector2/1, F_gear/1
  Constant/1 -> Cross Product/1
  Constant1/1 -> Cross Product1/1
  Constant2/1 -> Cross Product2/1
  Cross Product/1 -> Add1/1, Selector/1
  Cross Product1/1 -> Selector4/1, Add1/2
  Cross Product2/1 -> Add1/3
  Add1/1 -> M_gear/1
  [theta_eular] -> Scope6/1, MATLAB Function1/2(theta)
  [psi_eular] -> MATLAB Function1/3(psi)
  [theta_eular] -> MATLAB Function/2(theta)
  [phi_eular] -> MATLAB Function/1(phi)
  [psi_eular] -> MATLAB Function/3(psi)
  MATLAB Function/1(R_bg) -> Matrix Multiply3/1, Matrix Multiply2/1, Matrix Multiply/1
  [F_nose_g] -> Matrix Multiply/2
  [F_right_g] -> Matrix Multiply3/2
  [F_left_g] -> Matrix Multiply2/2
  Matrix Multiply2/1 -> Cross Product1/2
  Matrix Multiply3/1 -> Cross Product2/2
  Matrix Multiply/1 -> Cross Product/2
  Selector1/1 -> Scope/1
  Selector3/1 -> Scope2/1
  Selector2/1 -> Scope3/1
  Selector/1 -> Scope1/1
  Selector4/1 -> Scope7/1

== system A320_23b/Flight Phase Manager/Data Pre-processing/Subsystem1 ==
  判断条件 : Inport
  Compare To Constant15 : simulink/Logic and Bit Operations/Compare To Constant  relop=>=  const=1  OutDataTypeStr=boolean
  Constant1 : Constant
  Integrator1 : Integrator  ExternalReset=level
  Logical Operator6 : Logic  Operator=NOT  AllPortsSameDT=off  OutDataTypeStr=boolean
  out : Outport
  wires:
  判断条件/1 -> Logical Operator6/1
  Compare To Constant15/1 -> out/1
  Integrator1/1 -> Compare To Constant15/1
  Logical Operator6/1 -> Integrator1/2
  Constant1/1 -> Integrator1/1

== system A320_23b/Flight Phase Manager/Data Pre-processing/Subsystem2 ==
  判断条件 : Inport
  Compare To Constant15 : simulink/Logic and Bit Operations/Compare To Constant  relop=>=  const=1  OutDataTypeStr=boolean
  Constant1 : Constant
  Integrator1 : Integrator  ExternalReset=level
  Logical Operator6 : Logic  Operator=NOT  AllPortsSameDT=off  OutDataTypeStr=boolean
  out : Outport
  wires:
  Constant1/1 -> Integrator1/1
  Logical Operator6/1 -> Integrator1/2
  Integrator1/1 -> Compare To Constant15/1
  Compare To Constant15/1 -> out/1
  判断条件/1 -> Logical Operator6/1

== system A320_23b/Flight Phase Manager/Data Pre-processing/持续1秒 ==
  判断条件 : Inport
  Compare To Constant15 : simulink/Logic and Bit Operations/Compare To Constant  relop=>=  const=1  OutDataTypeStr=boolean
  Constant1 : Constant
  Integrator1 : Integrator  ExternalReset=level
  Logical Operator6 : Logic  Operator=NOT  AllPortsSameDT=off  OutDataTypeStr=boolean
  out : Outport
  wires:
  Constant1/1 -> Integrator1/1
  Logical Operator6/1 -> Integrator1/2
  Integrator1/1 -> Compare To Constant15/1
  Compare To Constant15/1 -> out/1
  判断条件/1 -> Logical Operator6/1

== system A320_23b/Flight Phase Manager/Data Pre-processing/持续1秒1 ==
  判断条件 : Inport
  Compare To Constant15 : simulink/Logic and Bit Operations/Compare To Constant  relop=>=  const=1  OutDataTypeStr=boolean
  Constant1 : Constant
  Integrator1 : Integrator  ExternalReset=level
  Logical Operator6 : Logic  Operator=NOT  AllPortsSameDT=off  OutDataTypeStr=boolean
  out : Outport
  wires:
  判断条件/1 -> Logical Operator6/1
  Compare To Constant15/1 -> out/1
  Integrator1/1 -> Compare To Constant15/1
  Logical Operator6/1 -> Integrator1/2
  Constant1/1 -> Integrator1/1

== system A320_23b/Guidance/起飞阶段/地面滑跑阶段(1) ==
  e_Y : Inport
  e_psi : Inport  Port=2
  r : Inport  Port=3
  Enable : EnablePort
  Bus Creator : BusCreator  Inputs=9
  Constant2 : Constant  Value=0
  Constant3 : Constant  Value=0
  Constant4 : Constant  Value=0.8
  下滑角占位 : Constant
  偏航角指令 : Subsystem
  刹车占位 : Constant  Value=0
  纵向过载占位 : Constant
  速度占位 : Constant
  高度占位 : Constant
  Cmd_Bus : Outport
  wires:
  Bus Creator/1 -> Cmd_Bus/1
  纵向过载占位/1 -> Bus Creator/1  "nz_cmd"
  Constant2/1 -> Bus Creator/2  "phi_cmd"
  偏航角指令/1(psi_cmd) -> Bus Creator/3  "psi_cmd"
  Constant3/1 -> Bus Creator/4  "theta_cmd"
  速度占位/1 -> Bus Creator/5  "V_cmd"
  Constant4/1 -> Bus Creator/6  "throttle_cmd"
  刹车占位/1 -> Bus Creator/7  "brake_cmd"
  下滑角占位/1 -> Bus Creator/8  "gamma"
  高度占位/1 -> Bus Creator/9  "H_cmd"
  e_Y/1 -> 偏航角指令/1(e_Y)
  e_psi/1 -> 偏航角指令/2(e_psi)
  r/1 -> 偏航角指令/3(r)

== system A320_23b/Guidance/起飞阶段/巡航阶段(5) ==
  Vwind_ground : Inport
  Va_safe : Inport  Port=2
  h_ALG : Inport  Port=3
  vzg : Inport  Port=4
  phi_eular : Inport  Port=5
  theta_eular : Inport  Port=6
  Enable : EnablePort
  Asin : Trigonometry  Operator=asin
  Bus Creator : BusCreator  Inputs=9
  Constant2 : Constant  Value=0
  Divide : Product  Inputs=*/
  Gain1 : Gain  Gain=-1
  Saturation2 : Saturate  UpperLimit=10*DH  LowerLimit=-10*DH
  Scope : Scope
  Selector : Selector  InputPortWidth=3  IndexOptions=Index vector (dialog)  Indices=2  OutputSizes=1
  Subsystem : Subsystem
  V_cmd : Constant  Value=V_cruise
  下滑角占位 : Constant
  俯仰角占位 : Constant  Value=0
  刹车占位 : Constant  Value=0
  油门占位 : Constant
  高度占位 : Constant
  Cmd_Bus : Outport
  wires:
  油门占位/1 -> Bus Creator/6  "throttle_cmd"
  Bus Creator/1 -> Cmd_Bus/1
  Constant2/1 -> Bus Creator/2  "phi_cmd"
  俯仰角占位/1 -> Bus Creator/4  "theta_cmd"
  V_cmd/1 -> Bus Creator/5  "V_cmd"
  Subsystem/1(nz_cmd) -> Scope/1, Bus Creator/1  "nz_cmd"
  下滑角占位/1 -> Bus Creator/8  "gamma"
  刹车占位/1 -> Bus Creator/7  "brake_cmd"
  Saturation2/1 -> Bus Creator/3  "psi_cmd"
  高度占位/1 -> Bus Creator/9  "H_cmd"
  Selector/1 -> Divide/1
  Divide/1 -> Asin/1
  Vwind_ground/1 -> Selector/1
  Asin/1 -> Gain1/1
  Va_safe/1 -> Divide/2
  Gain1/1 -> Saturation2/1
  h_ALG/1 -> Subsystem/1(h_ALG)
  vzg/1 -> Subsystem/2(vzg)
  phi_eular/1 -> Subsystem/3(phi_eular)
  theta_eular/1 -> Subsystem/4(theta_eular)

== system A320_23b/Guidance/起飞阶段/抬轮离地爬升阶段(2//3//4) ==
  Vwind_ground : Inport
  Va_safe : Inport  Port=2
  Enable : EnablePort
  Asin : Trigonometry  Operator=asin
  Bus Creator : BusCreator  Inputs=9
  Constant2 : Constant  Value=0
  Constant3 : Constant  Value=12*DH
  Constant4 : Constant
  Divide : Product  Inputs=*/
  Gain1 : Gain  Gain=-1
  Saturation2 : Saturate  UpperLimit=10*DH  LowerLimit=-10*DH
  Selector : Selector  InputPortWidth=3  IndexOptions=Index vector (dialog)  Indices=2  OutputSizes=1
  下滑角占位 : Constant
  刹车占位 : Constant  Value=0
  纵向过载占位 : Constant
  速度占位 : Constant
  高度占位 : Constant
  Cmd_Bus : Outport
  wires:
  Saturation2/1 -> Bus Creator/3  "psi_cmd"
  高度占位/1 -> Bus Creator/9  "H_cmd"
  刹车占位/1 -> Bus Creator/7  "brake_cmd"
  下滑角占位/1 -> Bus Creator/8  "gamma"
  Constant4/1 -> Bus Creator/6  "throttle_cmd"
  Constant3/1 -> Bus Creator/4  "theta_cmd"
  速度占位/1 -> Bus Creator/5  "V_cmd"
  Constant2/1 -> Bus Creator/2  "phi_cmd"
  纵向过载占位/1 -> Bus Creator/1  "nz_cmd"
  Bus Creator/1 -> Cmd_Bus/1
  Gain1/1 -> Saturation2/1
  Vwind_ground/1 -> Selector/1
  Asin/1 -> Gain1/1
  Divide/1 -> Asin/1
  Selector/1 -> Divide/1
  Va_safe/1 -> Divide/2

== system A320_23b/Guidance/降落阶段/拉平//接地//滑跑刹车阶段(11//12//13) ==
  Flight_Phase : Inport
  gamma_cmd : Inport  Port=2
  H_cmd : Inport  Port=3
  Vwind_ground : Inport  Port=4
  Va_safe : Inport  Port=5
  Enable : EnablePort
  Asin : Trigonometry  Operator=asin
  Bus Creator : BusCreator  Inputs=9
  Compare To Constant2 : simulink/Logic and Bit Operations/Compare To Constant  relop===  const=13  OutDataTypeStr=boolean
  Constant : Constant  Value=0
  Constant2 : Constant  Value=0
  Divide1 : Product  Inputs=*/
  Gain1 : Gain  Gain=-1
  Saturation2 : Saturate  UpperLimit=25*DH  LowerLimit=-25*DH
  Selector : Selector  InputPortWidth=3  IndexOptions=Index vector (dialog)  Indices=2  OutputSizes=1
  Switch3 : Switch  Criteria=u2 > Threshold  SaturateOnIntegerOverflow=off  InputSameDT=off
  theta占位 : Constant  Value=0
  刹车 : Constant
  拉平接地速度 : Constant  Value=V_flare
  油门 : Constant  Value=0
  纵向过载占位 : Constant
  Cmd_Bus : Outport
  wires:
  Bus Creator/1 -> Cmd_Bus/1
  theta占位/1 -> Bus Creator/4  "theta_cmd"
  Switch3/1 -> Bus Creator/7  "brake_cmd"
  油门/1 -> Bus Creator/6  "throttle_cmd"
  纵向过载占位/1 -> Bus Creator/1  "nz_cmd"
  Constant2/1 -> Bus Creator/2  "phi_cmd"
  Saturation2/1 -> Bus Creator/3  "psi_cmd"
  拉平接地速度/1 -> Bus Creator/5  "V_cmd"
  刹车/1 -> Switch3/1  "brake_cmd"
  Compare To Constant2/1 -> Switch3/2
  gamma_cmd/1 -> Bus Creator/8  "gamma"
  Constant/1 -> Switch3/3
  H_cmd/1 -> Bus Creator/9  "H_cmd"
  Gain1/1 -> Saturation2/1
  Flight_Phase/1 -> Compare To Constant2/1
  Asin/1 -> Gain1/1
  Vwind_ground/1 -> Selector/1
  Selector/1 -> Divide1/1
  Divide1/1 -> Asin/1
  Va_safe/1 -> Divide1/2

== system A320_23b/Guidance/降落阶段/进场//轨迹捕获阶段(6//7) ==
  Vwind_ground : Inport
  Va_safe : Inport  Port=2
  h_ALG : Inport  Port=3
  vzg : Inport  Port=4
  phi_eular : Inport  Port=5
  theta_eular : Inport  Port=6
  gamma_cmd : Inport  Port=7
  H_cmd : Inport  Port=8
  Enable : EnablePort
  Asin : Trigonometry  Operator=asin
  Bus Creator : BusCreator  Inputs=9
  Constant2 : Constant  Value=0
  Constant3 : Constant  Value=0
  Divide : Product  Inputs=*/
  Gain1 : Gain  Gain=-1
  Saturation2 : Saturate  UpperLimit=10*DH  LowerLimit=-10*DH
  Selector : Selector  InputPortWidth=3  IndexOptions=Index vector (dialog)  Indices=2  OutputSizes=1
  Subsystem : Subsystem
  V_cmd : Constant  Value=V_cruise
  刹车占位 : Constant  Value=0
  油门占位 : Constant
  Cmd_Bus : Outport
  wires:
  Gain1/1 -> Saturation2/1
  Vwind_ground/1 -> Selector/1
  Va_safe/1 -> Divide/2
  H_cmd/1 -> Bus Creator/9  "H_cmd"
  Saturation2/1 -> Bus Creator/3  "psi_cmd"
  gamma_cmd/1 -> Bus Creator/8  "gamma"
  V_cmd/1 -> Bus Creator/5  "V_cmd"
  Asin/1 -> Gain1/1
  Selector/1 -> Divide/1
  Divide/1 -> Asin/1
  刹车占位/1 -> Bus Creator/7  "brake_cmd"
  Constant3/1 -> Bus Creator/4  "theta_cmd"
  Bus Creator/1 -> Cmd_Bus/1
  油门占位/1 -> Bus Creator/6  "throttle_cmd"
  Constant2/1 -> Bus Creator/2  "phi_cmd"
  Subsystem/1(nz_cmd) -> Bus Creator/1  "nz_cmd"
  h_ALG/1 -> Subsystem/1(h_ALG)
  vzg/1 -> Subsystem/2(vzg)
  theta_eular/1 -> Subsystem/4(theta_eular)
  phi_eular/1 -> Subsystem/3(phi_eular)

== system A320_23b/Guidance/降落阶段/陡下滑//圆拉平//浅下滑阶段(8//9//10) ==
  Vwind_ground : Inport
  Va_safe : Inport  Port=2
  Flight_phase : Inport  Port=3
  h_ALG : Inport  Port=4
  vzg : Inport  Port=5
  phi_eular : Inport  Port=6
  theta_eular : Inport  Port=7
  gamma_cmd : Inport  Port=8
  H_cmd : Inport  Port=9
  Enable : EnablePort
  Asin : Trigonometry  Operator=asin
  Bus Creator : BusCreator  Inputs=9
  Compare To Constant : simulink/Logic and Bit Operations/Compare To Constant  relop===  const=8  OutDataTypeStr=boolean
  Constant2 : Constant  Value=0
  Constant3 : Constant  Value=12*DH
  Divide : Product  Inputs=*/
  Gain1 : Gain  Gain=-1
  Saturation2 : Saturate  UpperLimit=10*DH  LowerLimit=-10*DH
  Selector : Selector  InputPortWidth=3  IndexOptions=Index vector (dialog)  Indices=2  OutputSizes=1
  Subsystem : Subsystem
  Switch : Switch  Criteria=u2 > Threshold  SaturateOnIntegerOverflow=off  InputSameDT=off
  刹车占位 : Constant  Value=0
  圆拉平/浅下滑 : Constant  Value=V_shallow
  油门占位 : Constant
  陡下滑 : Constant  Value=V_app
  Cmd_Bus : Outport
  wires:
  Subsystem/1(nz_cmd) -> Bus Creator/1  "nz_cmd"
  Constant2/1 -> Bus Creator/2  "phi_cmd"
  油门占位/1 -> Bus Creator/6  "throttle_cmd"
  Bus Creator/1 -> Cmd_Bus/1
  Constant3/1 -> Bus Creator/4  "theta_cmd"
  刹车占位/1 -> Bus Creator/7  "brake_cmd"
  Divide/1 -> Asin/1
  Selector/1 -> Divide/1
  Asin/1 -> Gain1/1
  Saturation2/1 -> Bus Creator/3  "psi_cmd"
  H_cmd/1 -> Bus Creator/9  "H_cmd"
  Va_safe/1 -> Divide/2
  Vwind_ground/1 -> Selector/1
  Gain1/1 -> Saturation2/1
  陡下滑/1 -> Switch/1
  圆拉平/浅下滑/1 -> Switch/3
  Switch/1 -> Bus Creator/5  "V_cmd"
  Flight_phase/1 -> Compare To Constant/1
  Compare To Constant/1 -> Switch/2
  gamma_cmd/1 -> Bus Creator/8  "gamma"
  h_ALG/1 -> Subsystem/1(h_ALG)
  vzg/1 -> Subsystem/2(vzg)
  theta_eular/1 -> Subsystem/4(theta_eular)
  phi_eular/1 -> Subsystem/3(phi_eular)

== system A320_23b/controller1/1_Pitch_Ctrl/234俯仰角控制 ==
  theta_cmd : Inport
  theta : Inport  Port=2
  q : Inport  Port=3
  Gain : Gain  Gain=-2
  Gain1 : Gain  Gain=5
  Scope : Scope  NumInputPorts=2
  Sum : Sum  Inputs=|+-
  Sum2 : Sum  Inputs=|+-
  de_theta_rad : Outport
  wires:
  theta/1 -> Scope/2, Sum/2
  theta_cmd/1 -> Scope/1, Sum/1
  Sum/1 -> Gain1/1
  Gain1/1 -> Sum2/1
  q/1 -> Sum2/2
  Sum2/1 -> Gain/1
  Gain/1 -> de_theta_rad/1

== system A320_23b/controller1/1_Pitch_Ctrl/567三回路控制 ==
  nz_cmd : Inport
  nz : Inport  Port=2
  q : Inport  Port=3
  复位 : Inport  Port=4
  Constant1 : Constant  Value=Kn_pitch
  Constant2 : Constant  Value=K_alpha
  Constant3 : Constant  Value=Kw_pitch
  Integrator1 : Integrator  ExternalReset=level  LimitOutput=on  UpperSaturationLimit=0.10  LowerSaturationLimit=-0.10
  Product : Product
  Product1 : Product
  Product2 : Product
  Scope : Scope
  Subsystem : Subsystem
  Sum3 : Sum  Inputs=|+-
  Sum4 : Sum  Inputs=|+-
  Sum5 : Sum  Inputs=|+-
  de_nz_rad : Outport
  wires:
  q/1 -> Subsystem/1(q), Sum5/2
  nz_cmd/1 -> Sum3/1
  Constant2/1 -> Product1/1
  nz/1 -> Sum3/2
  Constant1/1 -> Product/1
  Sum4/1 -> Product1/2
  Constant3/1 -> Product2/1
  Sum3/1 -> Product/2
  Product/1 -> Integrator1/1
  Sum5/1 -> Product2/2
  Integrator1/1 -> Sum4/1
  Product1/1 -> Sum5/1
  Subsystem/1(alpha(伪攻角)) -> Sum4/2
  Product2/1 -> Scope/1, de_nz_rad/1
  复位/1 -> Integrator1/2

== system A320_23b/controller1/1_Pitch_Ctrl/89101112_着陆俯仰控制 ==
  Vg : Inport
  gamma : Inport  Port=2
  h_cmd : Inport  Port=3
  Add : Sum  Inputs=|+-
  Add1 : Sum  Inputs=|+-
  Add5 : Sum
  Add6 : Sum  Inputs=++--
  Compare To Constant : simulink/Logic and Bit Operations/Compare To Constant  relop===  const=8  OutDataTypeStr=boolean
  Gain : Gain  Gain=-1
  Gain1 : Gain  Gain=-0.84
  Gain2 : Gain  Gain=-0.45
  Gain3 : Gain  Gain=0.3
  Gain4 : Gain  Gain=-0.3
  Gain5 : Gain  Gain=1.0
  Gain6 : Gain  Gain=0.1
  Integrator : Integrator  ExternalReset=rising
  Product : Product
  SatDe : Saturate  UpperLimit=de_max  LowerLimit=de_min
  Scope : Scope  NumInputPorts=2
  Scope1 : Scope
  Sin : Trigonometry
  Subtract : Sum  Inputs=+-
  de(D) : Outport
  wires:
  Sin/1 -> Product/1
  Vg/1 -> Product/2
  Product/1 -> Add/1
  [vzg] -> Gain/1
  Gain/1 -> Add/2
  Add/1 -> Gain1/1
  h_cmd/1 -> Scope/1, Add1/1, Subtract/1
  [height] -> Add1/2, Scope/2, Subtract/2
  Add1/1 -> Gain2/1
  Gain4/1 -> Add6/3
  Gain3/1 -> Add6/4
  Add6/1 -> Gain5/1
  Gain5/1 -> Gain6/1, Add5/1
  Integrator/1 -> Add5/2
  Gain2/1 -> Add6/2
  Gain1/1 -> Add6/1
  Add5/1 -> SatDe/1
  SatDe/1 -> de(D)/1
  [q] -> Gain4/1
  Gain6/1 -> Integrator/1
  [nz] -> Gain3/1
  gamma/1 -> Sin/1
  Subtract/1 -> Scope1/1
  [Flight_Phase] -> Compare To Constant/1
  Compare To Constant/1 -> Integrator/2

== system A320_23b/controller1/2_Yaw_Ctrl/23456789101112段控制 ==
  Y : Inport
  psi : Inport  Port=2
  r : Inport  Port=3
  psi_cmd : Inport  Port=4
  Add : Sum  Inputs=+++
  Constant1 : Constant  Value=0
  Gain : Gain  Gain=-1.3
  Gain1 : Gain  Gain=0.2
  Gain2 : Gain  Gain=-0.05
  Gain3 : Gain  Gain=0.4
  Sum1 : Sum  Inputs=|+-
  Sum2 : Sum  Inputs=|++
  Sum3 : Sum  Inputs=|+-
  dr_cmd : Outport
  wires:
  Gain/1 -> Add/2
  Gain2/1 -> Sum2/1
  Constant1/1 -> Sum3/1
  [vyg] -> Gain1/1
  r/1 -> Gain3/1
  Gain3/1 -> Add/3
  Sum3/1 -> Gain2/1
  Sum2/1 -> Add/1
  Gain1/1 -> Sum2/2
  Add/1 -> dr_cmd/1
  psi/1 -> Sum1/2
  Sum1/1 -> Gain/1
  Y/1 -> Sum3/2
  psi_cmd/1 -> Sum1/1

== system A320_23b/6DOF-MODEL/AERO-PARAMETER/无量纲化角速率/Subsystem ==
  r : Inport
  Va : Inport  Port=2
  Constant4 : Constant  Value=b_ref
  Divide : Product  Inputs=*/
  Gain : Gain  Gain=2
  Product : Product
  r_hat : Outport
  wires:
  Va/1 -> Gain/1
  r/1 -> Product/1
  Constant4/1 -> Product/2
  Product/1 -> Divide/1
  Divide/1 -> r_hat/1
  Gain/1 -> Divide/2

== system A320_23b/6DOF-MODEL/AERO-PARAMETER/无量纲化角速率/Subsystem1 ==
  q : Inport
  Va : Inport  Port=2
  Constant4 : Constant  Value=c_ref
  Divide : Product  Inputs=*/
  Gain : Gain  Gain=2
  Product : Product
  Scope : Scope
  q_hat : Outport
  wires:
  Va/1 -> Gain/1
  q/1 -> Scope/1, Product/1
  Constant4/1 -> Product/2
  Product/1 -> Divide/1
  Divide/1 -> q_hat/1
  Gain/1 -> Divide/2

== system A320_23b/6DOF-MODEL/AERO-PARAMETER/无量纲化角速率/Subsystem2 ==
  p : Inport
  Va : Inport  Port=2
  Constant4 : Constant  Value=b_ref
  Divide : Product  Inputs=*/
  Gain : Gain  Gain=2
  Product : Product
  p_hat : Outport
  wires:
  Va/1 -> Gain/1
  p/1 -> Product/1
  Constant4/1 -> Product/2
  Product/1 -> Divide/1
  Divide/1 -> p_hat/1
  Gain/1 -> Divide/2
